simulink model "SRR_S_function_lastest"  (Simulink 8.5)
settings: Solver=ode23tb  StartTime=0.0  StopTime=0.5  FixedStep=5e-5  MinStep=1e-18  RelTol=10000  AbsTol=10000
values from neighbouring files (symbols this model uses):
  A = [1-b*Ts/J0,-Ts/J0;0,1]    [SRR_KF_RLS.m]
libraries: powerlib x5
settings Model: Creator=haoliang  LastModifiedBy=tradi
settings SolverCC: MaxConsecutiveZCs=1000000  MaxConsecutiveMinStep=1000
settings DebuggingCC: SolverPrmCheckMsg=warning  FcnCallInpInsideContextMsg=UseLocalSettings

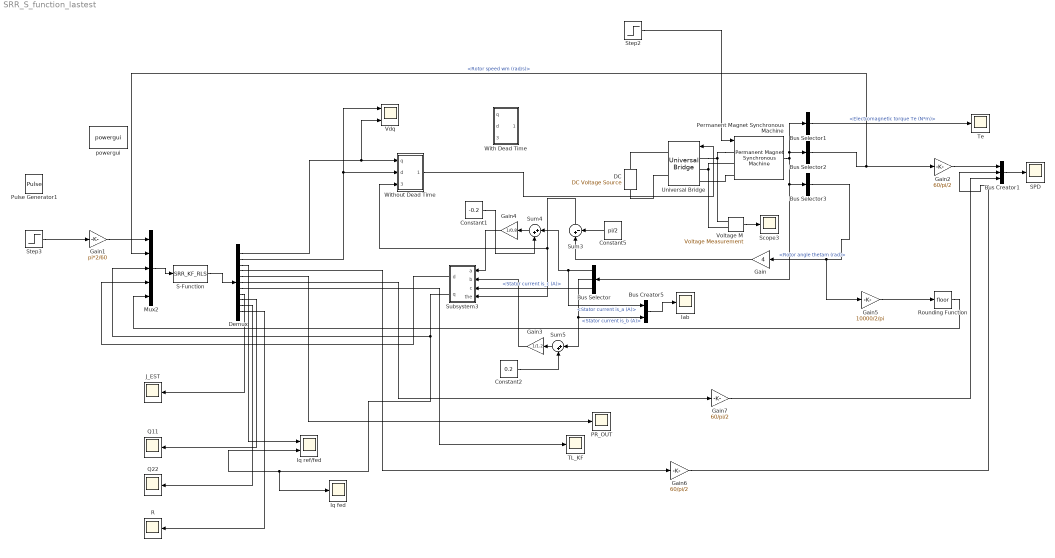
== system SRR_S_function_lastest ==
  Bus Creator1 : BusCreator  Inputs=3
  Bus Creator5 : BusCreator  Inputs=2
  Bus Selector : BusSelector  OutputSignals=Stator current is_a (A),Stator current is_b (A),Stator current is_c (A)
  Bus Selector1 : BusSelector  OutputSignals=Electromagnetic torque Te (N*m)
  Bus Selector2 : BusSelector  OutputSignals=Rotor speed wm (rad/s)
  Bus Selector3 : BusSelector  OutputSignals=Rotor angle thetam (rad)
  Constant1 : Constant  Value=-0.2  OutDataTypeStr=double
  Constant2 : Constant  Value=0.2  OutDataTypeStr=double
  Constant5 : Constant  Value=pi/2
  "DC " : powerlib/Electrical Sources/DC Voltage Source  Amplitude=300  Measurements=None
  Demux : Demux  Outputs=11
  Gain : Gain  Gain=4
  Gain1 : Gain  Gain=pi*2/60
  Gain2 : Gain  Gain=60/pi/2
  Gain3 : Gain  Gain=1/1.2
  Gain4 : Gain  Gain=1/0.8
  Gain5 : Gain  Gain=10000/2/pi
  Gain6 : Gain  Gain=60/pi/2
  Gain7 : Gain  Gain=60/pi/2
  Iab : Scope
      settings: YMin=-200  YMax=200  SaveName=TL4
  Iq fed : Scope
      settings: YMin=1.1  YMax=1.525  SaveName=IQfdb
  Iq ref/fed : Scope  NumInputPorts=2
      settings: YMin=1.1~0.8  YMax=1.525~1.5  SaveName=IQ1
  J_EST : Scope
      settings: YMin=1.0166  YMax=1.0184  SaveName=J_est
  Mux2 : Mux  Inputs=5
  PR_OUT : Scope
      settings: YMin=-0.0575  YMax=-0.0025  SaveName=Out_PR
  Permanent Magnet Synchronous Machine : powerlib/Machines/Permanent Magnet Synchronous Machine  NbPhases=3  FluxDistribution=Sinusoidal  RotorType=Salient-pole  MechanicalLoad=Torque Tm  PresetModel=No  ShowDetailedParameters=on  MeasurementBus=off  Resistance=0.45  Inductance=8.5e-3  dqInductances=[3.9e-3, 3.9e-3]  La=0.000835  MachineConstant=Voltage Constant (V_peak L-L / krpm)  Flux=0.0605  VoltageCst=43.8939  TorqueCst=0.363  Flat=120  Mechanical="[ 2*5.2e-4, 0.02,  4 ]"  PolePairs=4  InitialConditions=[0,0, 0,0]  InitialConditions5ph=[0 0 0 0 0 0]  TsPowergui=0  TsBlock=-1  RefAngle=90 degrees behind phase A axis (modified Park)
  Pulse Generator1 : DiscretePulseGenerator  PulseType=Time based  Amplitude=500  Period=0.1  PulseWidth=50
  Q11 : Scope
      settings: YMin=0.0260404  YMax=0.0260404  SaveName=Q11
  Q22 : Scope
      settings: YMin=1.1  YMax=1.525  SaveName=Q22
  R : Scope
      settings: TimeRange=0.5  YMin=0.95  YMax=1.05  SaveName=R
  Rounding Function : Rounding
  S-Function : S-Function  FunctionName=SRR_KF_RLS
  SPD : Scope
      settings: TimeRange=0.2  YMin=198.25  YMax=202.5  SaveName=SPD
  Scope3 : Scope
  Step2 : Step  Time=0.2  After=0  SampleTime=0
  Step3 : Step  Time=0  After=200  SampleTime=0
  Subsystem3 : Subsystem
  Sum3 : Sum  Inputs=|+-
  Sum4 : Sum  Inputs=|++
  Sum5 : Sum  Inputs=|++
  TL_KF : Scope
      settings: YMin=-4  YMax=13  SaveName=TL_KF
  Te : Scope
      settings: YMin=0.4  YMax=0.49  SaveName=ScopeData2
  Universal Bridge : powerlib/Power Electronics/Universal Bridge  Arms=3  SnubberResistance=1e5  SnubberCapacitance=inf  Device=Ideal Switches  Ron=1e-3  Lon=0  ForwardVoltages="[  0  0  ]"  ForwardVoltage=0  GTOparameters=[ 10e-6 , 20e-6 ]  IGBTparameters=[ 1e-6 , 2e-6 ]  Measurements=Device voltages  Measurements_2=None  converterType=Rectifier
  Vdq : Scope  NumInputPorts=2
      settings: YMin=-5~-5  YMax=5~5  SaveName=TL3
  Voltage M : powerlib/Measurements/Voltage Measurement  PhasorSimulation=off  OutputType=Complex  PSBequivalent=0
  With Dead Time : Subsystem
  Without Dead Time : Subsystem
  powergui : powerlib/powergui  Priority=1  SimulationMode=Continuous  SolverType=Tustin/Backward Euler (TBE)  SampleTime=1e-6  frequency=60  SPID=off  DisableSnubberDevices=off  DisableRonSwitches=off  DisableVfSwitches=off  SwTol=0  DisplayEquations=off  Interpol=off  methode=off  Ts=100  FunctionMessages=off  echomessages=off  HookPort=off  EnableUseOfTLC=off  x0status=blocks  frequencyindice=0  Pbase=100e6  ErrMax=1e-4  Iterations=50  UnitsV=kV  UnitsW=MW  buscounter=0  RestoreLinks=warning  ResistiveCurrentMeasurement=off  Frange=[0:2:500]  Ylog=off  Xlog=on  ShowGrid=off  save=off  variable=ZData  structure=SPD  ZoomFFT=off  StartTime=0.9  cycles=1  DisplayStyle=3  fundamental=200/15  FreqAxis=on  MaxFrequency=1000  frequencyindicesteady=1  RmsSteady=1  display=off
  wires:
  Permanent Magnet Synchronous Machine/1 -> Bus Selector3/1, Bus Selector/1, Bus Selector2/1, Bus Selector1/1
  Bus Selector2/1 -> Mux2/2, Gain2/1  "<Rotor speed wm (rad/s)>"
  Voltage M/1 -> Scope3/1
  Gain/1 -> Sum3/1
  Bus Selector3/1 -> Gain5/1, Gain/1  "<Rotor angle thetam (rad)>"
  Bus Selector/3 -> Subsystem3/3(c)  "<Stator current is_c (A)>"
  Subsystem3/1(d) -> Mux2/4
  Constant5/1 -> Sum3/2
  Bus Selector1/1 -> Te/1  "<Electromagnetic torque Te (N*m)>"
  Constant1/1 -> Sum4/2
  Constant2/1 -> Sum5/2
  Bus Selector/1 -> Bus Creator5/1, Sum4/1  "<Stator current is_a (A)>"
  Bus Selector/2 -> Sum5/1, Bus Creator5/2  "<Stator current is_b (A)>"
  Sum5/1 -> Gain3/1
  Gain3/1 -> Subsystem3/2(b)
  Sum4/1 -> Gain4/1
  Gain4/1 -> Subsystem3/1(a)
  Mux2/1 -> S-Function/1
  S-Function/1 -> Demux/1
  Gain1/1 -> Mux2/1
  Demux/3 -> Iq ref/fed/1
  Gain5/1 -> Rounding Function/1
  Demux/4 -> Gain6/1
  Rounding Function/1 -> Mux2/5
  Step2/1 -> Permanent Magnet Synchronous Machine/1
  Subsystem3/2(q) -> Mux2/3, Iq fed/1, Iq ref/fed/2
  Demux/2 -> Without Dead Time/2(d), Vdq/1
  Sum3/1 -> Without Dead Time/3(the), Subsystem3/4(the)
  Demux/1 -> Without Dead Time/1(q), Vdq/2
  Bus Creator5/1 -> Iab/1
  Demux/5 -> PR_OUT/1
  Gain6/1 -> Bus Creator1/2
  Gain2/1 -> Bus Creator1/1
  Bus Creator1/1 -> SPD/1
  Demux/6 -> Gain7/1
  Gain7/1 -> Bus Creator1/3
  Demux/7 -> TL_KF/1
  Demux/8 -> J_EST/1
  Demux/9 -> Q11/1
  Demux/10 -> Q22/1
  Demux/11 -> R/1
  Without Dead Time/1(Out1) -> Universal Bridge/1
  Step3/1 -> Gain1/1
  connections:
  Permanent Magnet Synchronous Machine/LConn1 -- Universal Bridge/LConn1 -- Voltage M/LConn1
  Universal Bridge/LConn2 -- Permanent Magnet Synchronous Machine/LConn2 -- Voltage M/LConn2
  "DC "/RConn1 -- Universal Bridge/RConn1
  "DC "/LConn1 -- Universal Bridge/RConn2
  Permanent Magnet Synchronous Machine/LConn3 -- Universal Bridge/LConn3

== system SRR_S_function_lastest/Subsystem3 ==
  a : Inport
  b : Inport  Port=2
  c : Inport  Port=3
  the : Inport  Port=4
  Bus Creator : BusCreator  Inputs=2
  Bus Creator1 : BusCreator  Inputs=3
  Fcn : Fcn  Expr=u[1]*cos(u[3])+u[2]*sin(u[3])
  Fcn1 : Fcn  Expr=u[2]*cos(u[3])-u[1]*sin(u[3])
  Gain1 : Gain  Gain=(1/3)^(0.5)
  Sum : Sum  Inputs=|+-
  beta1 : Fcn  Expr=u[1]+2*u[2]
  d : Outport
  q : Outport  Port=2
  wires:
  the/1 -> Sum/1
  Sum/1 -> Bus Creator1/3
  Bus Creator1/1 -> Fcn/1, Fcn1/1
  Fcn1/1 -> q/1
  Fcn/1 -> d/1
  Gain1/1 -> Bus Creator1/2
  Bus Creator/1 -> beta1/1
  beta1/1 -> Gain1/1
  b/1 -> Bus Creator/2
  a/1 -> Bus Creator/1, Bus Creator1/1

== system SRR_S_function_lastest/With Dead Time ==
  q : Inport
  d : Inport  Port=2
  the : Inport  Port=3
  Constant3 : Constant  Value=0.0001  OutDataTypeStr=double
  Constant4 : Constant  Value=300  OutDataTypeStr=double
  Data Type Conversion2 : DataTypeConversion  OutDataTypeStr=double
  Mux3 : Mux  Inputs=6
  Subsystem : Subsystem
  svpwm1 : Subsystem
  Out1 : Outport
  wires:
  d/1 -> Subsystem/2(d)
  q/1 -> Subsystem/1(q)
  Data Type Conversion2/1 -> Out1/1
  the/1 -> Subsystem/3(the)
  svpwm1/6(Opwm6) -> Mux3/6
  svpwm1/5(pwm5) -> Mux3/5
  svpwm1/4(pwm4) -> Mux3/4
  svpwm1/3(pwm3) -> Mux3/3
  svpwm1/2(pwm2) -> Mux3/2
  svpwm1/1(pwm1) -> Mux3/1
  Constant4/1 -> svpwm1/4(Udc)
  Constant3/1 -> svpwm1/3(tpwm)
  Subsystem/2(beta) -> svpwm1/2(vbeta)
  Subsystem/1(alpha) -> svpwm1/1(alpha)
  Mux3/1 -> Data Type Conversion2/1

== system SRR_S_function_lastest/Without Dead Time ==
  q : Inport
  d : Inport  Port=2
  the : Inport  Port=3
  Constant3 : Constant  Value=0.0001  OutDataTypeStr=double
  Constant4 : Constant  Value=300  OutDataTypeStr=double
  Data Type Conversion2 : DataTypeConversion  OutDataTypeStr=double
  Mux3 : Mux  Inputs=6
  Subsystem : Subsystem
  svpwm1 : Subsystem
  Out1 : Outport
  wires:
  d/1 -> Subsystem/2(d)
  q/1 -> Subsystem/1(q)
  Data Type Conversion2/1 -> Out1/1
  the/1 -> Subsystem/3(the)
  svpwm1/6(Opwm6) -> Mux3/6
  svpwm1/5(pwm5) -> Mux3/5
  svpwm1/4(pwm4) -> Mux3/4
  svpwm1/3(pwm3) -> Mux3/3
  svpwm1/2(pwm2) -> Mux3/2
  svpwm1/1(pwm1) -> Mux3/1
  Constant4/1 -> svpwm1/4(Udc)
  Constant3/1 -> svpwm1/3(tpwm)
  Subsystem/2(beta) -> svpwm1/2(vbeta)
  Subsystem/1(alpha) -> svpwm1/1(alpha)
  Mux3/1 -> Data Type Conversion2/1

== system SRR_S_function_lastest/With Dead Time/Subsystem ==
  q : Inport
  d : Inport  Port=2
  the : Inport  Port=3
  Bus Creator : BusCreator  Inputs=3
  Fcn : Fcn  Expr=cos(u[3])*u[2]-sin(u[3])*u[1]
  Fcn1 : Fcn  Expr=sin(u[3])*u[2]+cos(u[3])*u[1]
  Saturation : Saturate  UpperLimit=300  LowerLimit=-300
  Saturation1 : Saturate  UpperLimit=300  LowerLimit=-300
  alpha : Outport
  beta : Outport  Port=2
  wires:
  Saturation1/1 -> Bus Creator/2
  Saturation/1 -> Bus Creator/1
  Fcn1/1 -> beta/1
  Fcn/1 -> alpha/1
  Bus Creator/1 -> Fcn1/1, Fcn/1
  the/1 -> Bus Creator/3
  d/1 -> Saturation1/1
  q/1 -> Saturation/1

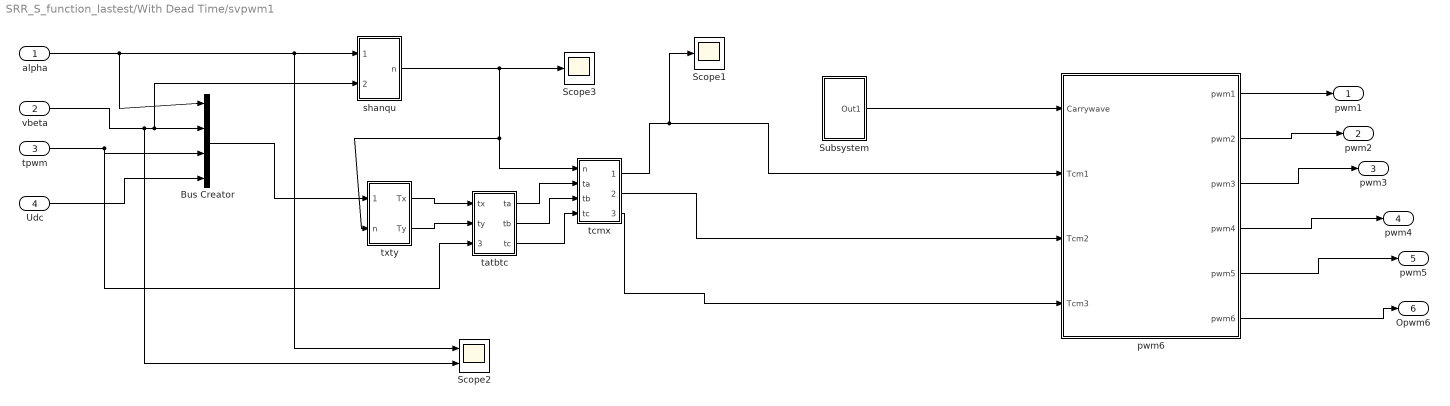
== system SRR_S_function_lastest/With Dead Time/svpwm1 ==
  alpha : Inport
  vbeta : Inport  Port=2
  tpwm : Inport  Port=3
  Udc : Inport  Port=4
  Bus Creator : BusCreator
  Scope1 : Scope
      settings: TimeRange=0.1  YMin=5e-006  YMax=4.5e-005  SaveName=ScopeData13
  Scope2 : Scope  NumInputPorts=2
      settings: TimeRange=0.1  YMin=2~-5  YMax=6~5  SaveName=ScopeData12
  Scope3 : Scope
      settings: TimeRange=0.1  YMin=2  YMax=6  SaveName=ScopeData3
  Subsystem : Subsystem
  pwm6 : Subsystem
  shanqu : Subsystem
  tatbtc : Subsystem
  tcmx : Subsystem
  txty : Subsystem
  pwm1 : Outport
  pwm2 : Outport  Port=2
  pwm3 : Outport  Port=3
  pwm4 : Outport  Port=4
  pwm5 : Outport  Port=5
  Opwm6 : Outport  Port=6
  wires:
  Bus Creator/1 -> txty/1(4gein)
  Udc/1 -> Bus Creator/4
  tpwm/1 -> Bus Creator/3, tatbtc/3(Tpwm)
  vbeta/1 -> Scope2/2, Bus Creator/2, shanqu/2(Vbeta)
  alpha/1 -> Scope2/1, shanqu/1(Valpha), Bus Creator/1
  shanqu/1(n) -> Scope3/1, txty/2(n), tcmx/1(n)
  tatbtc/3(tc) -> tcmx/4(tc)
  tatbtc/2(tb) -> tcmx/3(tb)
  tatbtc/1(ta) -> tcmx/2(ta)
  txty/2(Ty) -> tatbtc/2(ty)
  txty/1(Tx) -> tatbtc/1(tx)
  tcmx/3(tcm3) -> pwm6/4(Tcm3)
  tcmx/2(tcm2) -> pwm6/3(Tcm2)
  tcmx/1(tcm1) -> pwm6/2(Tcm1), Scope1/1
  Subsystem/1(Out1) -> pwm6/1(Carrywave)
  pwm6/1(pwm1) -> pwm1/1
  pwm6/2(pwm2) -> pwm2/1
  pwm6/3(pwm3) -> pwm3/1
  pwm6/4(pwm4) -> pwm4/1
  pwm6/5(pwm5) -> pwm5/1
  pwm6/6(pwm6) -> Opwm6/1

== system SRR_S_function_lastest/Without Dead Time/Subsystem ==
  q : Inport
  d : Inport  Port=2
  the : Inport  Port=3
  Bus Creator : BusCreator  Inputs=3
  Fcn : Fcn  Expr=cos(u[3])*u[2]-sin(u[3])*u[1]
  Fcn1 : Fcn  Expr=sin(u[3])*u[2]+cos(u[3])*u[1]
  Saturation : Saturate  UpperLimit=300  LowerLimit=-300
  Saturation1 : Saturate  UpperLimit=300  LowerLimit=-300
  alpha : Outport
  beta : Outport  Port=2
  wires:
  Saturation1/1 -> Bus Creator/2
  Saturation/1 -> Bus Creator/1
  Fcn1/1 -> beta/1
  Fcn/1 -> alpha/1
  Bus Creator/1 -> Fcn1/1, Fcn/1
  the/1 -> Bus Creator/3
  d/1 -> Saturation1/1
  q/1 -> Saturation/1

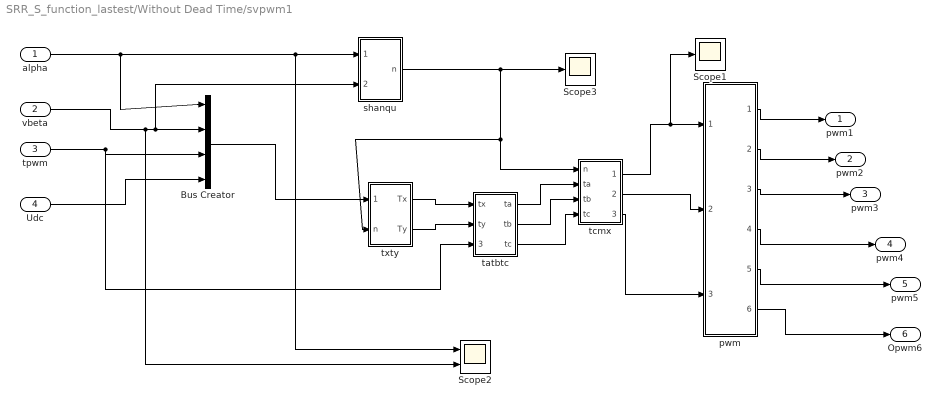
== system SRR_S_function_lastest/Without Dead Time/svpwm1 ==
  alpha : Inport
  vbeta : Inport  Port=2
  tpwm : Inport  Port=3
  Udc : Inport  Port=4
  Bus Creator : BusCreator
  Scope1 : Scope
      settings: TimeRange=0.1  YMin=5e-006  YMax=4.5e-005  SaveName=ScopeData13
  Scope2 : Scope  NumInputPorts=2
      settings: TimeRange=0.1  YMin=2~-5  YMax=6~5  SaveName=ScopeData12
  Scope3 : Scope
      settings: TimeRange=0.1  YMin=2  YMax=6  SaveName=ScopeData3
  pwm : Subsystem
  shanqu : Subsystem
  tatbtc : Subsystem
  tcmx : Subsystem
  txty : Subsystem
  pwm1 : Outport
  pwm2 : Outport  Port=2
  pwm3 : Outport  Port=3
  pwm4 : Outport  Port=4
  pwm5 : Outport  Port=5
  Opwm6 : Outport  Port=6
  wires:
  pwm/6(pwm6) -> Opwm6/1
  pwm/4(pwm4) -> pwm4/1
  pwm/2(pwm2) -> pwm2/1
  pwm/5(pwm5) -> pwm5/1
  pwm/3(pwm3) -> pwm3/1
  pwm/1(pwm1) -> pwm1/1
  Bus Creator/1 -> txty/1(4gein)
  Udc/1 -> Bus Creator/4
  tpwm/1 -> Bus Creator/3, tatbtc/3(Tpwm)
  vbeta/1 -> Scope2/2, Bus Creator/2, shanqu/2(Vbeta)
  alpha/1 -> Scope2/1, shanqu/1(Valpha), Bus Creator/1
  shanqu/1(n) -> Scope3/1, txty/2(n), tcmx/1(n)
  tatbtc/3(tc) -> tcmx/4(tc)
  tatbtc/2(tb) -> tcmx/3(tb)
  tatbtc/1(ta) -> tcmx/2(ta)
  txty/2(Ty) -> tatbtc/2(ty)
  txty/1(Tx) -> tatbtc/1(tx)
  tcmx/3(tcm3) -> pwm/3(cm33)
  tcmx/2(tcm2) -> pwm/2(tcm2)
  tcmx/1(tcm1) -> Scope1/1, pwm/1(tcm1)

== system SRR_S_function_lastest/With Dead Time/svpwm1/Subsystem ==
  Constant : Constant
  Integrator : Integrator
  Pulse Generator : DiscretePulseGenerator  PulseType=Time based  Amplitude=2  Period=0.0001  PulseWidth=50
  Scope : Scope  NumInputPorts=2
      settings: YMin=-5~-5  YMax=5~5
  Sum : Sum  Inputs=|+-
  Out1 : Outport
  wires:
  Integrator/1 -> Scope/1, Out1/1
  Sum/1 -> Integrator/1
  Constant/1 -> Sum/2
  Pulse Generator/1 -> Scope/2, Sum/1

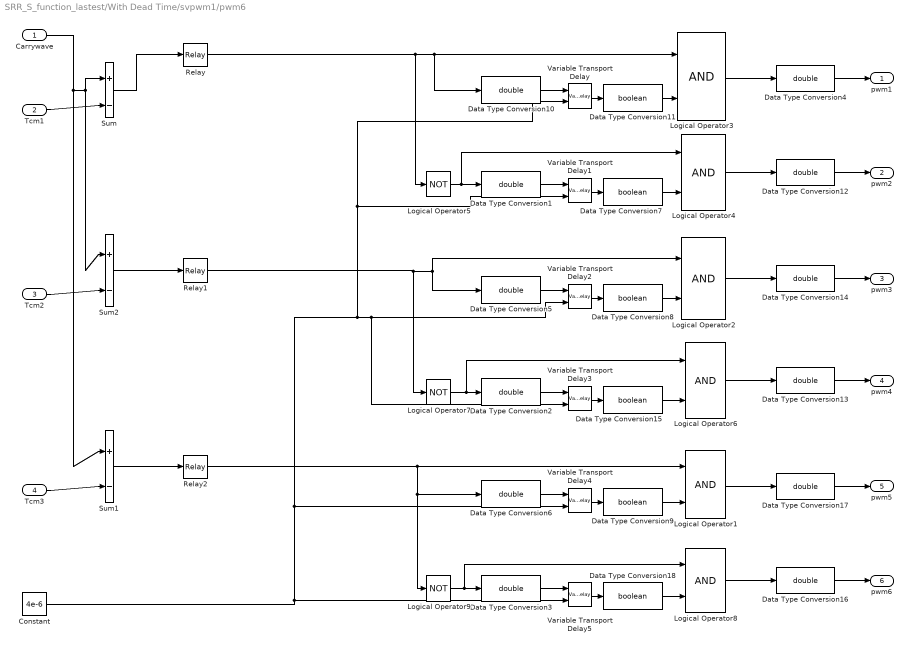
== system SRR_S_function_lastest/With Dead Time/svpwm1/pwm6 ==
  Carrywave : Inport
  Tcm1 : Inport  Port=2
  Tcm2 : Inport  Port=3
  Tcm3 : Inport  Port=4
  Constant : Constant  Value=4e-6
  Data Type Conversion{1..6,10,12..14,16..17} (12 alike) : DataTypeConversion  OutDataTypeStr=double
  Data Type Conversion{7..9,11,15,18} (6 alike) : DataTypeConversion  OutDataTypeStr=boolean
  Logical Operator{1..4,6,8} (6 alike) : Logic  AllPortsSameDT=off  OutDataTypeStr=boolean
  Logical Operator5 : Logic  Operator=NOT  AllPortsSameDT=off  OutDataTypeStr=boolean
  Logical Operator7 : Logic  Operator=NOT  AllPortsSameDT=off  OutDataTypeStr=boolean
  Logical Operator9 : Logic  Operator=NOT  AllPortsSameDT=off  OutDataTypeStr=boolean
  Relay : Relay
  Relay1 : Relay
  Relay2 : Relay
  Sum : Sum  Inputs=|+-
  Sum1 : Sum  Inputs=|+-
  Sum2 : Sum  Inputs=|+-
  Variable Transport Delay{,2..5} (5 alike) : VariableTransportDelay  VariableDelayType=Variable transport delay  MaximumDelay=10
  Variable Transport Delay1 : VariableTransportDelay  MaximumDelay=10
  pwm1 : Outport
  pwm2 : Outport  Port=2
  pwm3 : Outport  Port=3
  pwm4 : Outport  Port=4
  pwm5 : Outport  Port=5
  pwm6 : Outport  Port=6
  wires:
  Logical Operator8/1 -> Data Type Conversion16/1
  Data Type Conversion18/1 -> Logical Operator8/2
  Variable Transport Delay5/1 -> Data Type Conversion18/1
  Data Type Conversion3/1 -> Variable Transport Delay5/1
  Data Type Conversion16/1 -> pwm6/1
  Logical Operator9/1 -> Data Type Conversion3/1, Logical Operator8/1
  Logical Operator1/1 -> Data Type Conversion17/1
  Data Type Conversion9/1 -> Logical Operator1/2
  Variable Transport Delay4/1 -> Data Type Conversion9/1
  Data Type Conversion6/1 -> Variable Transport Delay4/1
  Data Type Conversion17/1 -> pwm5/1
  Relay2/1 -> Logical Operator1/1, Logical Operator9/1, Data Type Conversion6/1
  Logical Operator6/1 -> Data Type Conversion13/1
  Data Type Conversion15/1 -> Logical Operator6/2
  Variable Transport Delay3/1 -> Data Type Conversion15/1
  Data Type Conversion2/1 -> Variable Transport Delay3/1
  Data Type Conversion13/1 -> pwm4/1
  Logical Operator7/1 -> Data Type Conversion2/1, Logical Operator6/1
  Logical Operator2/1 -> Data Type Conversion14/1
  Data Type Conversion8/1 -> Logical Operator2/2
  Variable Transport Delay2/1 -> Data Type Conversion8/1
  Data Type Conversion5/1 -> Variable Transport Delay2/1
  Data Type Conversion14/1 -> pwm3/1
  Relay1/1 -> Logical Operator7/1, Data Type Conversion5/1, Logical Operator2/1
  Logical Operator4/1 -> Data Type Conversion12/1
  Data Type Conversion7/1 -> Logical Operator4/2
  Variable Transport Delay1/1 -> Data Type Conversion7/1
  Data Type Conversion1/1 -> Variable Transport Delay1/1
  Data Type Conversion12/1 -> pwm2/1
  Logical Operator5/1 -> Logical Operator4/1, Data Type Conversion1/1
  Logical Operator3/1 -> Data Type Conversion4/1
  Data Type Conversion11/1 -> Logical Operator3/2
  Variable Transport Delay/1 -> Data Type Conversion11/1
  Data Type Conversion10/1 -> Variable Transport Delay/1
  Constant/1 -> Variable Transport Delay3/2, Variable Transport Delay2/2, Variable Transport Delay1/2, Variable Transport Delay/2, Variable Transport Delay4/2, Variable Transport Delay5/2
  Data Type Conversion4/1 -> pwm1/1
  Carrywave/1 -> Sum1/1, Sum2/1, Sum/1
  Sum/1 -> Relay/1
  Sum2/1 -> Relay1/1
  Sum1/1 -> Relay2/1
  Relay/1 -> Logical Operator5/1, Data Type Conversion10/1, Logical Operator3/1
  Tcm2/1 -> Sum2/2
  Tcm3/1 -> Sum1/2
  Tcm1/1 -> Sum/2

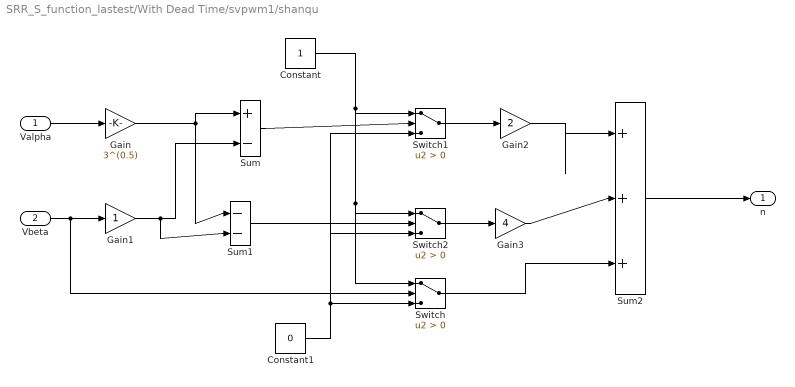
== system SRR_S_function_lastest/With Dead Time/svpwm1/shanqu ==
  Valpha : Inport
  Vbeta : Inport  Port=2
  Constant : Constant
  Constant1 : Constant  Value=0
  Gain : Gain  Gain=3^(0.5)
  Gain1 : Gain
  Gain2 : Gain  Gain=2
  Gain3 : Gain  Gain=4
  Sum : Sum  Inputs=|+-
  Sum1 : Sum  Inputs=|--
  Sum2 : Sum  Inputs=|+++
  Switch : Switch  Criteria=u2 > Threshold
  Switch1 : Switch  Criteria=u2 > Threshold
  Switch2 : Switch  Criteria=u2 > Threshold
  n : Outport
  wires:
  Gain3/1 -> Sum2/2
  Switch/1 -> Sum2/3
  Sum2/1 -> n/1
  Switch2/1 -> Gain3/1
  Switch1/1 -> Gain2/1
  Gain2/1 -> Sum2/1
  Sum1/1 -> Switch2/2
  Constant/1 -> Switch/1, Switch2/1, Switch1/1
  Sum/1 -> Switch1/2
  Constant1/1 -> Switch2/3, Switch1/3, Switch/3
  Gain1/1 -> Sum1/2, Sum/2
  Gain/1 -> Sum1/1, Sum/1
  Vbeta/1 -> Gain1/1, Switch/2
  Valpha/1 -> Gain/1

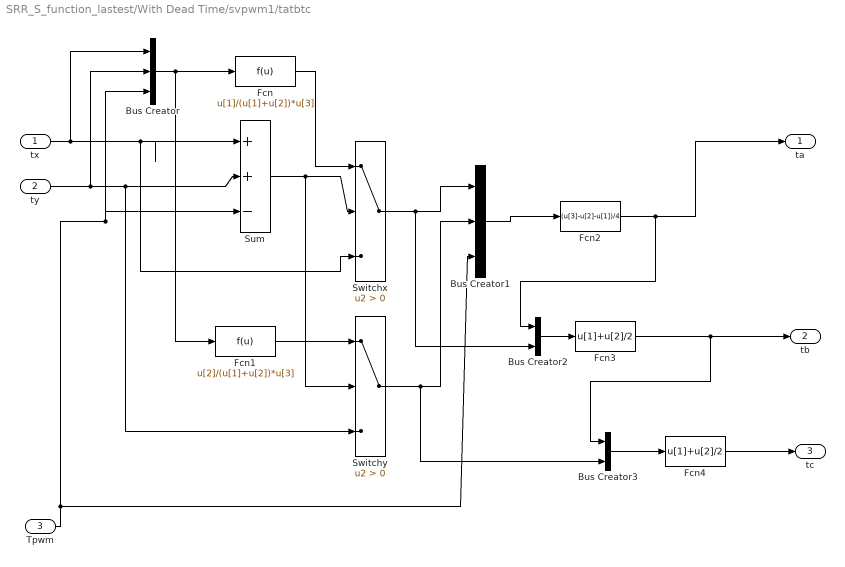
== system SRR_S_function_lastest/With Dead Time/svpwm1/tatbtc ==
  tx : Inport
  ty : Inport  Port=2
  Tpwm : Inport  Port=3
  Bus Creator : BusCreator  Inputs=3
  Bus Creator1 : BusCreator  Inputs=3
  Bus Creator2 : BusCreator  Inputs=2
  Bus Creator3 : BusCreator  Inputs=2
  Fcn : Fcn  Expr=u[1]/(u[1]+u[2])*u[3]
  Fcn1 : Fcn  Expr=u[2]/(u[1]+u[2])*u[3]
  Fcn2 : Fcn  Expr=(u[3]-u[2]-u[1])/4
  Fcn3 : Fcn  Expr=u[1]+u[2]/2
  Fcn4 : Fcn  Expr=u[1]+u[2]/2
  Sum : Sum  Inputs=|++-
  Switchx : Switch  Criteria=u2 > Threshold
  Switchy : Switch  Criteria=u2 > Threshold
  ta : Outport
  tb : Outport  Port=2
  tc : Outport  Port=3
  wires:
  Fcn4/1 -> tc/1
  Bus Creator3/1 -> Fcn4/1
  Fcn3/1 -> Bus Creator3/1, tb/1
  Bus Creator2/1 -> Fcn3/1
  Fcn2/1 -> Bus Creator2/1, ta/1
  Bus Creator1/1 -> Fcn2/1
  Switchy/1 -> Bus Creator3/2, Bus Creator1/2
  Switchx/1 -> Bus Creator2/2, Bus Creator1/1
  Fcn1/1 -> Switchy/1
  Fcn/1 -> Switchx/1
  Bus Creator/1 -> Fcn1/1, Fcn/1
  Sum/1 -> Switchy/2, Switchx/2
  Tpwm/1 -> Sum/3, Bus Creator/3, Bus Creator1/3
  ty/1 -> Bus Creator/2, Sum/2, Switchy/3
  tx/1 -> Bus Creator/1, Sum/1, Switchx/3

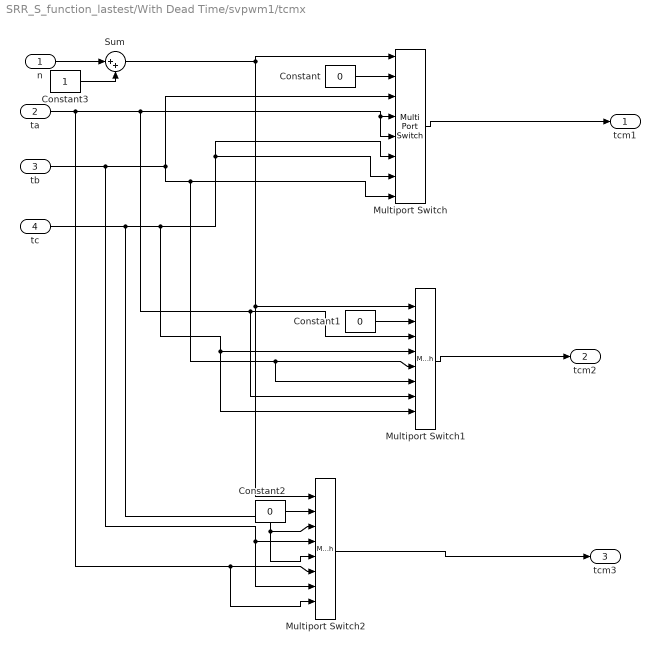
== system SRR_S_function_lastest/With Dead Time/svpwm1/tcmx ==
  n : Inport
  ta : Inport  Port=2
  tb : Inport  Port=3
  tc : Inport  Port=4
  Constant : Constant  Value=0
  Constant1 : Constant  Value=0
  Constant2 : Constant  Value=0
  Constant3 : Constant
  Multiport Switch : MultiPortSwitch  Inputs=7
  Multiport Switch1 : MultiPortSwitch  Inputs=7
  Multiport Switch2 : MultiPortSwitch  Inputs=7
  Sum : Sum  Inputs=|++
  tcm1 : Outport
  tcm2 : Outport  Port=2
  tcm3 : Outport  Port=3
  wires:
  Sum/1 -> Multiport Switch2/1, Multiport Switch1/1, Multiport Switch/1
  Constant3/1 -> Sum/2
  n/1 -> Sum/1
  Constant2/1 -> Multiport Switch2/2
  Constant1/1 -> Multiport Switch1/2
  Constant/1 -> Multiport Switch/2
  Multiport Switch2/1 -> tcm3/1
  Multiport Switch1/1 -> tcm2/1
  Multiport Switch/1 -> tcm1/1
  tc/1 -> Multiport Switch/6, Multiport Switch/7, Multiport Switch1/4, Multiport Switch1/8, Multiport Switch2/3, Multiport Switch2/5
  ta/1 -> Multiport Switch/4, Multiport Switch/5, Multiport Switch1/3, Multiport Switch1/7, Multiport Switch2/6, Multiport Switch2/8
  tb/1 -> Multiport Switch/3, Multiport Switch/8, Multiport Switch1/5, Multiport Switch1/6, Multiport Switch2/4, Multiport Switch2/7

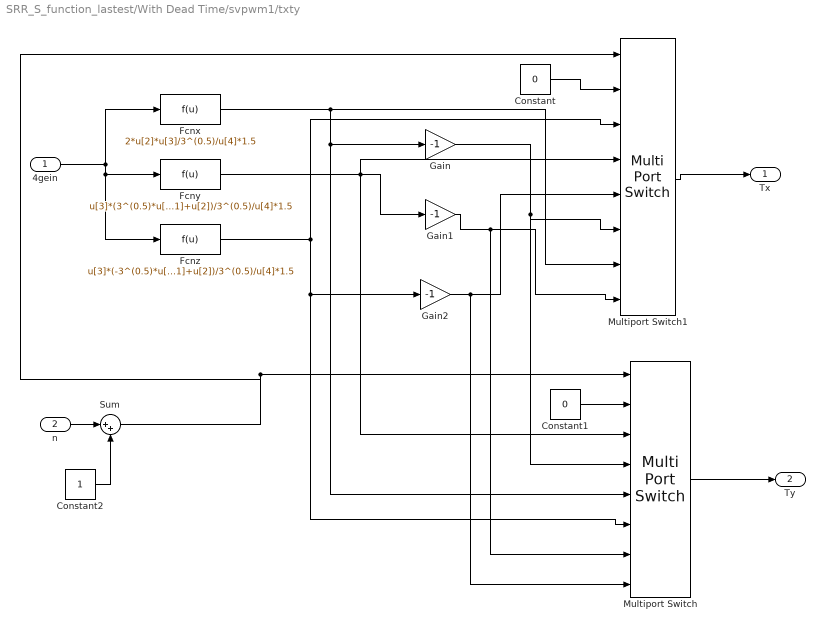
== system SRR_S_function_lastest/With Dead Time/svpwm1/txty ==
  4gein : Inport
  n : Inport  Port=2
  Constant : Constant  Value=0
  Constant1 : Constant  Value=0
  Constant2 : Constant
  Fcnx : Fcn  Expr=2*u[2]*u[3]/3^(0.5)/u[4]*1.5
  Fcny : Fcn  Expr=u[3]*(3^(0.5)*u[1]+u[2])/3^(0.5)/u[4]*1.5
  Fcnz : Fcn  Expr=u[3]*(-3^(0.5)*u[1]+u[2])/3^(0.5)/u[4]*1.5
  Gain : Gain  Gain=-1
  Gain1 : Gain  Gain=-1
  Gain2 : Gain  Gain=-1
  Multiport Switch : MultiPortSwitch  Inputs=7
  Multiport Switch1 : MultiPortSwitch  Inputs=7
  Sum : Sum  Inputs=|++
  Tx : Outport
  Ty : Outport  Port=2
  wires:
  Sum/1 -> Multiport Switch1/1, Multiport Switch/1
  Constant2/1 -> Sum/2
  n/1 -> Sum/1
  Constant1/1 -> Multiport Switch/2
  Constant/1 -> Multiport Switch1/2
  Multiport Switch/1 -> Ty/1
  Multiport Switch1/1 -> Tx/1
  Gain1/1 -> Multiport Switch/7, Multiport Switch1/8
  Fcny/1 -> Multiport Switch/3, Multiport Switch1/4, Gain1/1
  Gain/1 -> Multiport Switch/4, Multiport Switch1/6
  Fcnx/1 -> Multiport Switch1/7, Multiport Switch/5, Gain/1
  Gain2/1 -> Multiport Switch/8, Multiport Switch1/5
  Fcnz/1 -> Multiport Switch1/3, Multiport Switch/6, Gain2/1
  4gein/1 -> Fcnx/1, Fcny/1, Fcnz/1

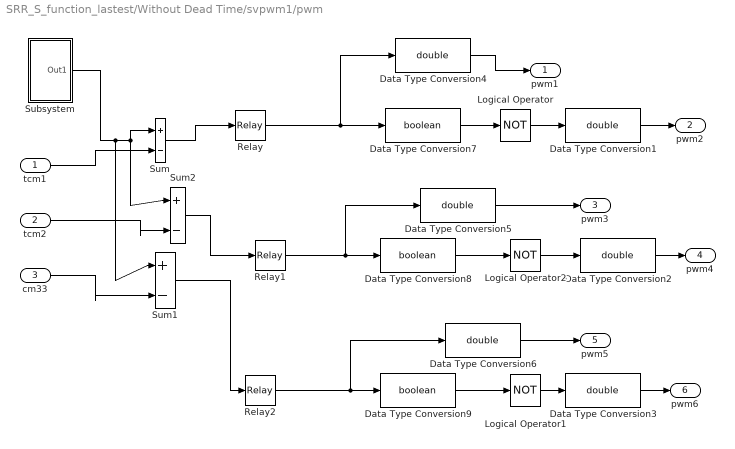
== system SRR_S_function_lastest/Without Dead Time/svpwm1/pwm ==
  tcm1 : Inport
  tcm2 : Inport  Port=2
  cm33 : Inport  Port=3
  Data Type Conversion{1..6} (6 alike) : DataTypeConversion  OutDataTypeStr=double
  Data Type Conversion7 : DataTypeConversion  OutDataTypeStr=boolean
  Data Type Conversion8 : DataTypeConversion  OutDataTypeStr=boolean
  Data Type Conversion9 : DataTypeConversion  OutDataTypeStr=boolean
  Logical Operator : Logic  Operator=NOT  AllPortsSameDT=off  OutDataTypeStr=boolean
  Logical Operator1 : Logic  Operator=NOT  AllPortsSameDT=off  OutDataTypeStr=boolean
  Logical Operator2 : Logic  Operator=NOT  AllPortsSameDT=off  OutDataTypeStr=boolean
  Relay : Relay
  Relay1 : Relay
  Relay2 : Relay
  Subsystem : Subsystem
  Sum : Sum  Inputs=|+-
  Sum1 : Sum  Inputs=|+-
  Sum2 : Sum  Inputs=|+-
  pwm1 : Outport
  pwm2 : Outport  Port=2
  pwm3 : Outport  Port=3
  pwm4 : Outport  Port=4
  pwm5 : Outport  Port=5
  pwm6 : Outport  Port=6
  wires:
  Data Type Conversion9/1 -> Logical Operator1/1
  Data Type Conversion8/1 -> Logical Operator2/1
  Data Type Conversion7/1 -> Logical Operator/1
  Data Type Conversion6/1 -> pwm5/1
  Data Type Conversion5/1 -> pwm3/1
  Data Type Conversion4/1 -> pwm1/1
  Data Type Conversion3/1 -> pwm6/1
  Logical Operator1/1 -> Data Type Conversion3/1
  Data Type Conversion2/1 -> pwm4/1
  Logical Operator2/1 -> Data Type Conversion2/1
  Data Type Conversion1/1 -> pwm2/1
  Logical Operator/1 -> Data Type Conversion1/1
  Subsystem/1(Out1) -> Sum1/1, Sum2/1, Sum/1
  Sum/1 -> Relay/1
  Sum2/1 -> Relay1/1
  Sum1/1 -> Relay2/1
  Relay/1 -> Data Type Conversion7/1, Data Type Conversion4/1
  Relay1/1 -> Data Type Conversion8/1, Data Type Conversion5/1
  Relay2/1 -> Data Type Conversion9/1, Data Type Conversion6/1
  tcm2/1 -> Sum2/2
  cm33/1 -> Sum1/2
  tcm1/1 -> Sum/2

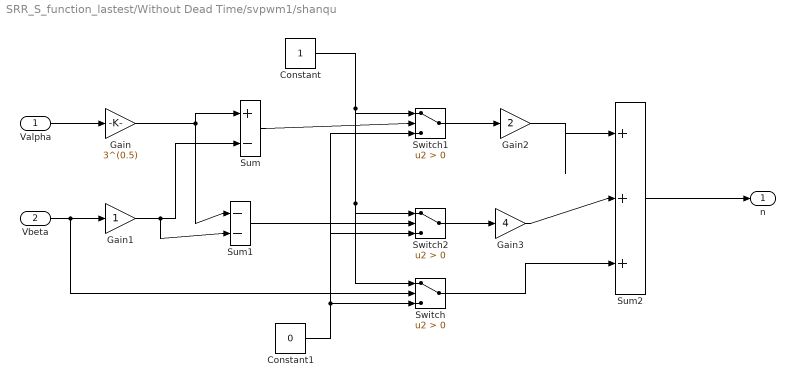
== system SRR_S_function_lastest/Without Dead Time/svpwm1/shanqu ==
  Valpha : Inport
  Vbeta : Inport  Port=2
  Constant : Constant
  Constant1 : Constant  Value=0
  Gain : Gain  Gain=3^(0.5)
  Gain1 : Gain
  Gain2 : Gain  Gain=2
  Gain3 : Gain  Gain=4
  Sum : Sum  Inputs=|+-
  Sum1 : Sum  Inputs=|--
  Sum2 : Sum  Inputs=|+++
  Switch : Switch  Criteria=u2 > Threshold
  Switch1 : Switch  Criteria=u2 > Threshold
  Switch2 : Switch  Criteria=u2 > Threshold
  n : Outport
  wires:
  Gain3/1 -> Sum2/2
  Switch/1 -> Sum2/3
  Sum2/1 -> n/1
  Switch2/1 -> Gain3/1
  Switch1/1 -> Gain2/1
  Gain2/1 -> Sum2/1
  Sum1/1 -> Switch2/2
  Constant/1 -> Switch/1, Switch2/1, Switch1/1
  Sum/1 -> Switch1/2
  Constant1/1 -> Switch2/3, Switch1/3, Switch/3
  Gain1/1 -> Sum1/2, Sum/2
  Gain/1 -> Sum1/1, Sum/1
  Vbeta/1 -> Gain1/1, Switch/2
  Valpha/1 -> Gain/1

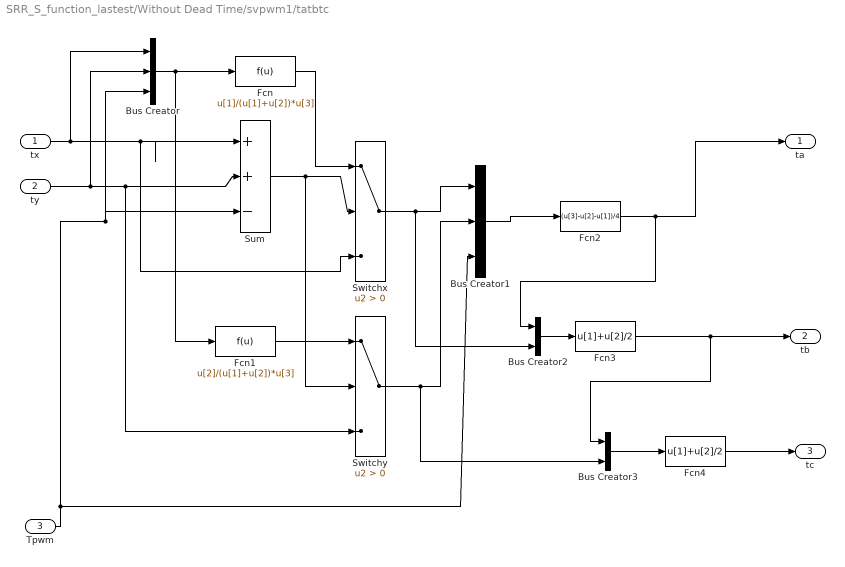
== system SRR_S_function_lastest/Without Dead Time/svpwm1/tatbtc ==
  tx : Inport
  ty : Inport  Port=2
  Tpwm : Inport  Port=3
  Bus Creator : BusCreator  Inputs=3
  Bus Creator1 : BusCreator  Inputs=3
  Bus Creator2 : BusCreator  Inputs=2
  Bus Creator3 : BusCreator  Inputs=2
  Fcn : Fcn  Expr=u[1]/(u[1]+u[2])*u[3]
  Fcn1 : Fcn  Expr=u[2]/(u[1]+u[2])*u[3]
  Fcn2 : Fcn  Expr=(u[3]-u[2]-u[1])/4
  Fcn3 : Fcn  Expr=u[1]+u[2]/2
  Fcn4 : Fcn  Expr=u[1]+u[2]/2
  Sum : Sum  Inputs=|++-
  Switchx : Switch  Criteria=u2 > Threshold
  Switchy : Switch  Criteria=u2 > Threshold
  ta : Outport
  tb : Outport  Port=2
  tc : Outport  Port=3
  wires:
  Fcn4/1 -> tc/1
  Bus Creator3/1 -> Fcn4/1
  Fcn3/1 -> Bus Creator3/1, tb/1
  Bus Creator2/1 -> Fcn3/1
  Fcn2/1 -> Bus Creator2/1, ta/1
  Bus Creator1/1 -> Fcn2/1
  Switchy/1 -> Bus Creator3/2, Bus Creator1/2
  Switchx/1 -> Bus Creator2/2, Bus Creator1/1
  Fcn1/1 -> Switchy/1
  Fcn/1 -> Switchx/1
  Bus Creator/1 -> Fcn1/1, Fcn/1
  Sum/1 -> Switchy/2, Switchx/2
  Tpwm/1 -> Sum/3, Bus Creator/3, Bus Creator1/3
  ty/1 -> Bus Creator/2, Sum/2, Switchy/3
  tx/1 -> Bus Creator/1, Sum/1, Switchx/3

== system SRR_S_function_lastest/Without Dead Time/svpwm1/tcmx ==
  n : Inport
  ta : Inport  Port=2
  tb : Inport  Port=3
  tc : Inport  Port=4
  Constant : Constant  Value=0
  Constant1 : Constant  Value=0
  Constant2 : Constant  Value=0
  Constant3 : Constant
  Multiport Switch : MultiPortSwitch  Inputs=7
  Multiport Switch1 : MultiPortSwitch  Inputs=7
  Multiport Switch2 : MultiPortSwitch  Inputs=7
  Sum : Sum  Inputs=|++
  tcm1 : Outport
  tcm2 : Outport  Port=2
  tcm3 : Outport  Port=3
  wires:
  Sum/1 -> Multiport Switch2/1, Multiport Switch1/1, Multiport Switch/1
  Constant3/1 -> Sum/2
  n/1 -> Sum/1
  Constant2/1 -> Multiport Switch2/2
  Constant1/1 -> Multiport Switch1/2
  Constant/1 -> Multiport Switch/2
  Multiport Switch2/1 -> tcm3/1
  Multiport Switch1/1 -> tcm2/1
  Multiport Switch/1 -> tcm1/1
  tc/1 -> Multiport Switch/6, Multiport Switch/7, Multiport Switch1/4, Multiport Switch1/8, Multiport Switch2/3, Multiport Switch2/5
  ta/1 -> Multiport Switch/4, Multiport Switch/5, Multiport Switch1/3, Multiport Switch1/7, Multiport Switch2/6, Multiport Switch2/8
  tb/1 -> Multiport Switch/3, Multiport Switch/8, Multiport Switch1/5, Multiport Switch1/6, Multiport Switch2/4, Multiport Switch2/7

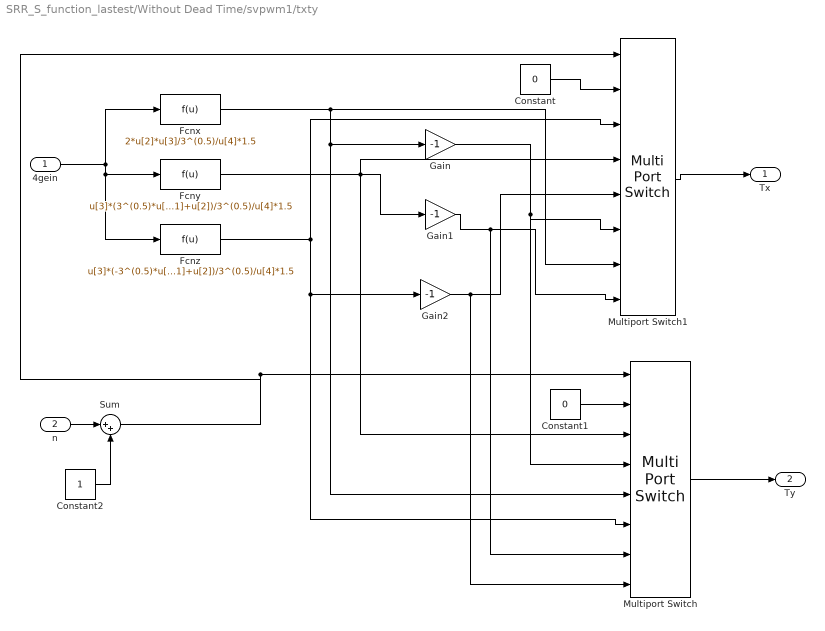
== system SRR_S_function_lastest/Without Dead Time/svpwm1/txty ==
  4gein : Inport
  n : Inport  Port=2
  Constant : Constant  Value=0
  Constant1 : Constant  Value=0
  Constant2 : Constant
  Fcnx : Fcn  Expr=2*u[2]*u[3]/3^(0.5)/u[4]*1.5
  Fcny : Fcn  Expr=u[3]*(3^(0.5)*u[1]+u[2])/3^(0.5)/u[4]*1.5
  Fcnz : Fcn  Expr=u[3]*(-3^(0.5)*u[1]+u[2])/3^(0.5)/u[4]*1.5
  Gain : Gain  Gain=-1
  Gain1 : Gain  Gain=-1
  Gain2 : Gain  Gain=-1
  Multiport Switch : MultiPortSwitch  Inputs=7
  Multiport Switch1 : MultiPortSwitch  Inputs=7
  Sum : Sum  Inputs=|++
  Tx : Outport
  Ty : Outport  Port=2
  wires:
  Sum/1 -> Multiport Switch1/1, Multiport Switch/1
  Constant2/1 -> Sum/2
  n/1 -> Sum/1
  Constant1/1 -> Multiport Switch/2
  Constant/1 -> Multiport Switch1/2
  Multiport Switch/1 -> Ty/1
  Multiport Switch1/1 -> Tx/1
  Gain1/1 -> Multiport Switch/7, Multiport Switch1/8
  Fcny/1 -> Multiport Switch/3, Multiport Switch1/4, Gain1/1
  Gain/1 -> Multiport Switch/4, Multiport Switch1/6
  Fcnx/1 -> Multiport Switch1/7, Multiport Switch/5, Gain/1
  Gain2/1 -> Multiport Switch/8, Multiport Switch1/5
  Fcnz/1 -> Multiport Switch1/3, Multiport Switch/6, Gain2/1
  4gein/1 -> Fcnx/1, Fcny/1, Fcnz/1

== system SRR_S_function_lastest/Without Dead Time/svpwm1/pwm/Subsystem ==
  Constant : Constant
  Integrator : Integrator
  Pulse Generator : DiscretePulseGenerator  PulseType=Time based  Amplitude=2  Period=0.0001  PulseWidth=50
  Scope : Scope  NumInputPorts=2
      settings: YMin=-5~-5  YMax=5~5
  Sum : Sum  Inputs=|+-
  Out1 : Outport
  wires:
  Integrator/1 -> Scope/1, Out1/1
  Sum/1 -> Integrator/1
  Constant/1 -> Sum/2
  Pulse Generator/1 -> Scope/2, Sum/1
